simulink model "quadrotor_mode"  (R2023b)
settings: Solver=VariableStepAuto  StartTime=0.0  StopTime=10.0  RelTol=1e-3
model workspace (MAT data in the model file):
  K = 1
  KR = 1
  Kd = 1
undefined symbols (not defined in the file or in its folder): Earth, WGS84
libraries: shared6dof x1, aerolib6dof2 x1
settings Model: Creator=lakshmikanth  LastModifiedBy=lakshmikanth

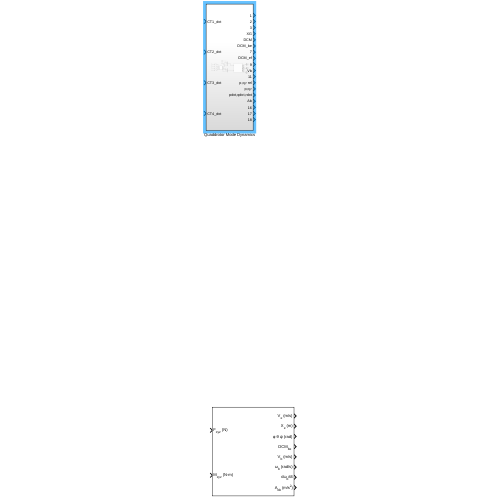
[thumbnail: Simulink's stored preview of the top-level diagram]
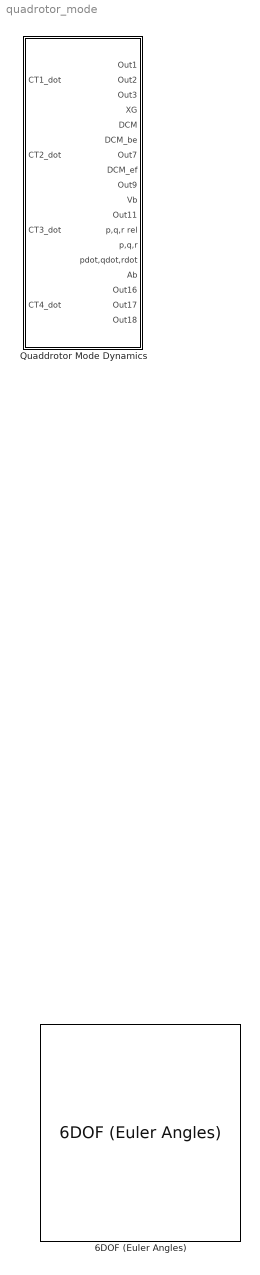
== system quadrotor_mode ==
  6DOF (Euler Angles) : shared6dof/6DOF (Euler Angles)  units=Metric (MKS)  mtype=Fixed  rep=Euler Angles  xme_0=[0 0 0]  Vm_0=[0 0 0]  eul_0=[0 0 0]  pm_0=[0 0 0]  mass_0=1.0  mass_e=0.5  mass_f=2.0  inertia=eye(3)  inertia_e=eye(3)  inertia_f=2*eye(3)  k_quat=1.0  vre_flag=on  abi_flag=off  aMode=0  xme_statename=''  Vm_statename=''  eul_statename=''  quat_statename=''  pm_statename=''  mass_statename=''
  Quaddrotor Mode Dynamics : Subsystem

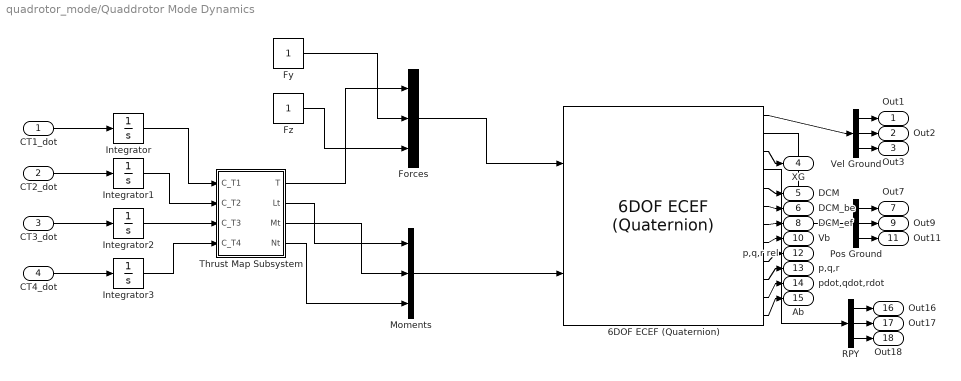
== system quadrotor_mode/Quaddrotor Mode Dynamics ==
  CT1_dot : Inport
  CT2_dot : Inport  Port=2
  CT3_dot : Inport  Port=3
  CT4_dot : Inport  Port=4
  6DOF ECEF (Quaternion) : aerolib6dof2/6DOF ECEF (Quaternion)  units=Metric (MKS)  mtype=Fixed  xg_0=[0 0 0]  Vm_0=[0 0 0]  eul_0=[0 0 0]  pm_0=[0 0 0]  mass_0=1.0  mass_e=0.5  mass_f=2.0  inertia=eye(3)  inertia_e=eye(3)  inertia_f=2*eye(3)  vre_flag=on  abi_flag=off  ptype=Earth (WGS84)  R=6378137  F=1/298.257223563  w_E=7292115e-11  angle_in=Internal  LPM0=0  quat_statename=''  pm_statename=''  Vm_statename=''  posfixedframe_statename=''  posinertial_statename=''  LPM_statename=''  mass_statename=''
  Forces : Mux  Inputs=3
  Fy : Constant
  Fz : Constant
  Integrator{,1..3} (4 alike) : Integrator
  Moments : Mux  Inputs=3
  Pos Ground : Demux  Outputs=3
  RPY : Demux  Outputs=3
  Thrust Map Subsystem : Subsystem
  Vel Ground : Demux  Outputs=3
  Out1 : Outport
  Out2 : Outport  Port=2
  Out3 : Outport  Port=3
  XG : Outport  Port=4
  DCM : Outport  Port=5
  DCM_be : Outport  Port=6
  Out7 : Outport  Port=7
  DCM_ef : Outport  Port=8
  Out9 : Outport  Port=9
  Vb : Outport  Port=10
  Out11 : Outport  Port=11
  p,q,r rel : Outport  Port=12
  p,q,r : Outport  Port=13
  pdot,qdot,rdot : Outport  Port=14
  Ab : Outport  Port=15
  Out16 : Outport  Port=16
  Out17 : Outport  Port=17
  Out18 : Outport  Port=18
  wires:
  Integrator/1 -> Thrust Map Subsystem/1(C_T1)
  6DOF ECEF (Quaternion)/6 -> DCM_be/1
  6DOF ECEF (Quaternion)/1 -> Vel Ground/1
  Fz/1 -> Forces/3
  RPY/3 -> Out18/1
  Pos Ground/1 -> Out7/1
  6DOF ECEF (Quaternion)/2 -> Pos Ground/1
  6DOF ECEF (Quaternion)/5 -> DCM/1
  6DOF ECEF (Quaternion)/12 -> Ab/1
  Thrust Map Subsystem/2(Lt) -> Moments/1
  Pos Ground/2 -> Out9/1
  Integrator3/1 -> Thrust Map Subsystem/4(C_T4)
  6DOF ECEF (Quaternion)/3 -> XG/1
  Thrust Map Subsystem/1(T) -> Forces/1
  Vel Ground/1 -> Out1/1
  Integrator2/1 -> Thrust Map Subsystem/3(C_T3)
  6DOF ECEF (Quaternion)/7 -> DCM_ef/1
  6DOF ECEF (Quaternion)/9 -> p,q,r rel/1
  6DOF ECEF (Quaternion)/4 -> RPY/1
  6DOF ECEF (Quaternion)/11 -> pdot,qdot,rdot/1
  Moments/1 -> 6DOF ECEF (Quaternion)/2
  RPY/2 -> Out17/1
  6DOF ECEF (Quaternion)/10 -> p,q,r/1
  Thrust Map Subsystem/4(Nt) -> Moments/3
  Pos Ground/3 -> Out11/1
  Fy/1 -> Forces/2
  Vel Ground/2 -> Out2/1
  Forces/1 -> 6DOF ECEF (Quaternion)/1
  RPY/1 -> Out16/1
  Vel Ground/3 -> Out3/1
  Integrator1/1 -> Thrust Map Subsystem/2(C_T2)
  Thrust Map Subsystem/3(Mt) -> Moments/2
  6DOF ECEF (Quaternion)/8 -> Vb/1
  CT1_dot/1 -> Integrator/1
  CT2_dot/1 -> Integrator1/1
  CT3_dot/1 -> Integrator2/1
  CT4_dot/1 -> Integrator3/1

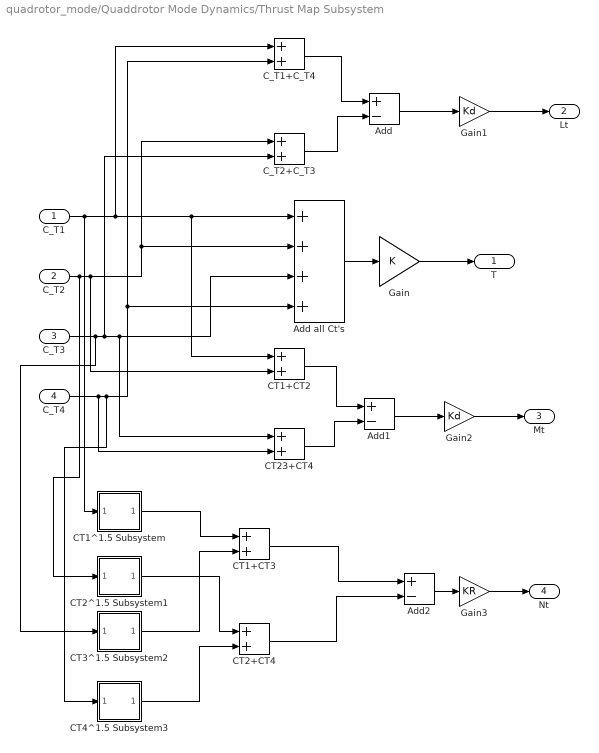
== system quadrotor_mode/Quaddrotor Mode Dynamics/Thrust Map Subsystem ==
  C_T1 : Inport
  C_T2 : Inport  Port=2
  C_T3 : Inport  Port=3
  C_T4 : Inport  Port=4
  Add : Sum  Inputs=+-
  Add all Ct's : Sum  Inputs=++++
  Add1 : Sum  Inputs=+-
  Add2 : Sum  Inputs=+-
  CT1+CT2 : Sum
  CT1+CT3 : Sum
  CT1^1.5 Subsystem : Subsystem
  CT2+CT4 : Sum
  CT23+CT4 : Sum
  CT2^1.5 Subsystem1 : Subsystem
  CT3^1.5 Subsystem2 : Subsystem
  CT4^1.5 Subsystem3 : Subsystem
  C_T1+C_T4 : Sum
  C_T2+C_T3 : Sum
  Gain : Gain  Gain=K
  Gain1 : Gain  Gain=Kd
  Gain2 : Gain  Gain=Kd
  Gain3 : Gain  Gain=KR
  T : Outport
  Lt : Outport  Port=2
  Mt : Outport  Port=3
  Nt : Outport  Port=4
  wires:
  CT23+CT4/1 -> Add1/2
  CT1+CT2/1 -> Add1/1
  Gain1/1 -> Lt/1
  Add1/1 -> Gain2/1
  Gain2/1 -> Mt/1
  Gain3/1 -> Nt/1
  CT3^1.5 Subsystem2/1(Out1) -> CT1+CT3/2
  CT1^1.5 Subsystem/1(Out1) -> CT1+CT3/1
  CT1+CT3/1 -> Add2/1
  Add2/1 -> Gain3/1
  C_T1+C_T4/1 -> Add/1
  C_T2/1 -> CT2^1.5 Subsystem1/1(Input), CT1+CT2/2, C_T2+C_T3/1, Add all Ct's/2
  C_T3/1 -> CT3^1.5 Subsystem2/1(Input), C_T2+C_T3/2, CT23+CT4/1, Add all Ct's/3
  C_T4/1 -> CT23+CT4/2, CT4^1.5 Subsystem3/1(Input), C_T1+C_T4/2, Add all Ct's/4
  C_T2+C_T3/1 -> Add/2
  C_T1/1 -> CT1^1.5 Subsystem/1(Input), CT1+CT2/1, Add all Ct's/1, C_T1+C_T4/1
  CT2^1.5 Subsystem1/1(Out1) -> CT2+CT4/1
  CT4^1.5 Subsystem3/1(Out1) -> CT2+CT4/2
  CT2+CT4/1 -> Add2/2
  Add all Ct's/1 -> Gain/1
  Add/1 -> Gain1/1
  Gain/1 -> T/1

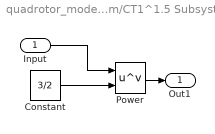
== system quadrotor_mode/Quaddrotor Mode Dynamics/Thrust Map Subsystem/CT1^1.5 Subsystem ==
  Input : Inport
  Constant : Constant  Value=3/2
  Power : Math  Operator=pow
  Out1 : Outport
  wires:
  Constant/1 -> Power/2
  Input/1 -> Power/1
  Power/1 -> Out1/1

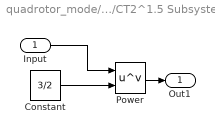
== system quadrotor_mode/Quaddrotor Mode Dynamics/Thrust Map Subsystem/CT2^1.5 Subsystem1 ==
  Input : Inport
  Constant : Constant  Value=3/2
  Power : Math  Operator=pow
  Out1 : Outport
  wires:
  Constant/1 -> Power/2
  Input/1 -> Power/1
  Power/1 -> Out1/1

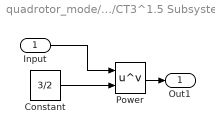
== system quadrotor_mode/Quaddrotor Mode Dynamics/Thrust Map Subsystem/CT3^1.5 Subsystem2 ==
  Input : Inport
  Constant : Constant  Value=3/2
  Power : Math  Operator=pow
  Out1 : Outport
  wires:
  Constant/1 -> Power/2
  Input/1 -> Power/1
  Power/1 -> Out1/1

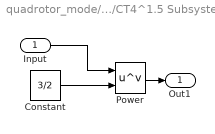
== system quadrotor_mode/Quaddrotor Mode Dynamics/Thrust Map Subsystem/CT4^1.5 Subsystem3 ==
  Input : Inport
  Constant : Constant  Value=3/2
  Power : Math  Operator=pow
  Out1 : Outport
  wires:
  Constant/1 -> Power/2
  Input/1 -> Power/1
  Power/1 -> Out1/1
